simulink model "HydraulicLinearMotorArm"  (R2024a)
settings: Solver=FixedStepAuto  StartTime=0.0  StopTime=inf  MaxStep=0.033333333333333333  RelTol=1e-3  EnableMultiTasking=on
libraries: arduinolib x9, SignalEditorBlockLib x6, arduinosensorlib x2, simulink_extras x1, aerolibanimutils x1
settings Model: ExtModeTrigDuration=2  Creator=Akbar  LastModifiedBy=Akbar
settings SolverCC: AutoInsertRateTranBlk=on
settings OptimizationCC: EnhancedBackFolding=on  PassReuseOutputArgsAs=Individual arguments  ZeroExternalMemoryAtStartup=off  ZeroInternalMemoryAtStartup=off  MaxStackSize=64  OptimizeBlockOrder=speed  DifferentSizesBufferReuse=on  OptimizationCustomize=off  EfficientTunableParamExpr=on
settings DebuggingCC: ParameterTunabilityLossMsg=error
settings HardwareCC: ProdBitPerPointer=32  ProdBitPerSizeT=32  ProdBitPerPtrDiffT=32  ProdLargestAtomicInteger=Long  ProdLargestAtomicFloat=Double  ProdWordSize=32  ProdHWDeviceType=ARM Compatible->ARM Cortex
settings SFSimCC: MATLABDynamicMemAlloc=off
settings RTWCC: Description=Embedded Coder  SystemTargetFile=ert.tlc  HardwareBoard=ESP32-WROOM(Arduino Compatible)  TLCOptions="-aInlineSetEventsForThisBaseRateFcn=TLC_FALSE -aSuppressMultiTaskScheduler=TLC_FALSE  -aRateBasedStepFcn=0"  TemplateMakefile=ert_default_tmf  Toolchain=ESP32  BuildConfiguration=Faster Runs
settings CodeAppCC: ForceParamTrailComments=on  IgnoreCustomStorageClasses=off  OperatorAnnotations=on  SimulinkDataObjDesc=on  SFDataObjDesc=on  InsertBlockDesc=on
settings ERTTargetCC: SupportContinuousTime=on  SupportVariableSizeSignals=on  ExtModeTransport=3  ExtModeStaticAlloc=on  ExtModeAutomaticAllocSize=off  ExtModeStaticAllocSize=65536  ExtModeMexFile=ext_xcp  ExtModeIntrfLevel=Level2 - Open

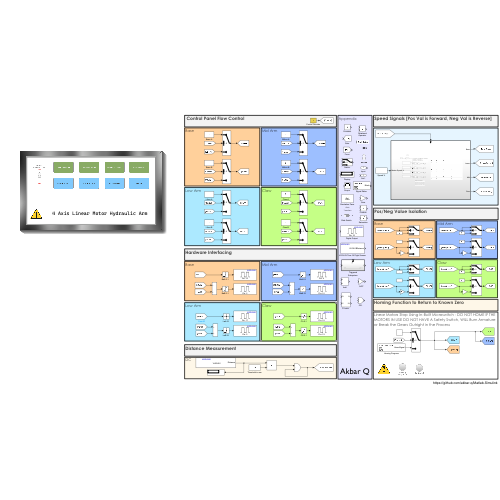
[thumbnail: Simulink's stored preview of the top-level diagram]
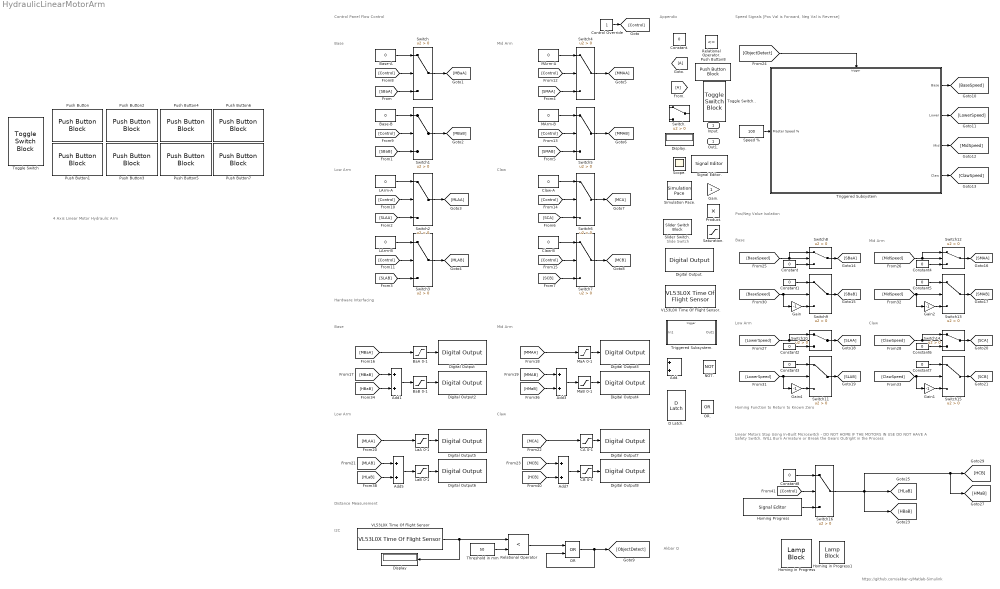
== system HydraulicLinearMotorArm ==
  note: https://github.com/akbar-q/Matlab-Simulink
  note: Akbar Q
  note: 4 Axis Linear Motor Hydraulic Arm
  note: Slide Switch
  note: Appendix
  note: Control Panel Flow Control
  note: Base
  note: Low Arm
  note: Mid Arm
  note: Claw
  note: Claw
  note: Hardware Interfacing
  note: Low Arm
  note: Mid Arm
  note: Base
  note: Distance Measurement
  note: I2C
  note: Speed Signals [Pos Val is Forward, Neg Val is Reverse]
  note: Pos/Neg Value Isolation
  note: Claw
  note: Base
  note: Low Arm
  note: Mid Arm
  note: Homing Function to Return to Known Zero
  note: Linear Motors Stop Using In-Built Microswitch - DO NOT HOME IF THE
      | MOTORS IN USE DO NOT HAVE A Safety Switch, WILL Burn Armature
      | or Break the Gears Outright in the Process
  Input. : Inport
  Add. : Sum
  Add{1,3,5,7} (4 alike) : Sum
  BaA 0-1 : Saturate  UpperLimit=1  LowerLimit=0
  BaB 0-1 : Saturate  UpperLimit=1  LowerLimit=0
  Base-A : Constant  Value=0
  Base-B : Constant  Value=0
  CA 0-1 : Saturate  UpperLimit=1  LowerLimit=0
  CB 0-1 : Saturate  UpperLimit=1  LowerLimit=0
  Claw-A : Constant  Value=0
  Claw-B : Constant  Value=0
  Constant{,1..8} (9 alike) : Constant  Value=0
  Constant. : Constant  Value=0
  Control Override : Constant
  D Latch. : simulink_extras/Flip Flops/D Latch
  Digital Output : arduinolib/Digital Output  pinNumber=15  Direction=output  blockPlatform=arduino
  Digital Output. : arduinolib/Digital Output  pinNumber=33  Direction=output  blockPlatform=arduino
  Digital Output2 : arduinolib/Digital Output  pinNumber=2  Direction=output  blockPlatform=arduino
  Digital Output3 : arduinolib/Digital Output  pinNumber=4  Direction=output  blockPlatform=arduino
  Digital Output4 : arduinolib/Digital Output  pinNumber=16  Direction=output  blockPlatform=arduino
  Digital Output5 : arduinolib/Digital Output  pinNumber=17  Direction=output  blockPlatform=arduino
  Digital Output6 : arduinolib/Digital Output  pinNumber=5  Direction=output  blockPlatform=arduino
  Digital Output7 : arduinolib/Digital Output  pinNumber=18  Direction=output  blockPlatform=arduino
  Digital Output8 : arduinolib/Digital Output  pinNumber=19  Direction=output  blockPlatform=arduino
  Display : Display
  Display. : Display
  From. : From
  Gain{,1..2,4} (4 alike) : Gain  Gain=-1
  Gain. : Gain
  Goto. : Goto
  Homing Progress : SignalEditorBlockLib/Signal Editor  FileName=C:\Users\Akbar\Cloud-Drive_maa32ocd@bolton.ac.uk\Hobby Projects\GitHub Repos\Matlab-Simulink\ESP32-Arm-4DOF-Binary\SpeedSignals\HomeSignal.mat  ActiveScenario=HomingFunction  ActiveSignal=HomeSignal  IsBus=off  OutputBusObjectStr=Bus: BusObject  SampleTime=0  Interpolate=off  ZeroCross=off  OutputAfterFinalValue=Setting to zero  Unit=inherit  PreserveSignalName=on  ApplySigPropsToAllScenarios=on  ApplySigPropsToAllSignals=off
  Homing in Progress : LampBlock  LabelPosition=Bottom
  Homing in Progress1 : LampBlock  LabelPosition=Bottom
  LArm-A : Constant  Value=0
  LArm-B : Constant  Value=0
  LaA 0-1 : Saturate  UpperLimit=1  LowerLimit=0
  LaB 0-1 : Saturate  UpperLimit=1  LowerLimit=0
  MArm-A : Constant  Value=0
  MArm-B : Constant  Value=0
  MaA 0-1 : Saturate  UpperLimit=1  LowerLimit=0
  MaB 0-1 : Saturate  UpperLimit=1  LowerLimit=0
  NOT. : Logic  Operator=NOT  IconShape=distinctive  AllPortsSameDT=off  OutDataTypeStr=boolean
  OR : Logic  Operator=OR  IconShape=distinctive  AllPortsSameDT=off  OutDataTypeStr=boolean
  OR. : Logic  Operator=OR  IconShape=distinctive  AllPortsSameDT=off  OutDataTypeStr=boolean
  Product. : Product
  Push Button : PushButtonBlock  ButtonText=Base Clockwise  OffValue=0.000000
  Push Button1 : PushButtonBlock  ButtonText=Base AntiClock  OffValue=0.000000
  Push Button2 : PushButtonBlock  ButtonText=Low Arm Forward  OffValue=0.000000
  Push Button3 : PushButtonBlock  ButtonText=Low Arm Back  OffValue=0.000000
  Push Button4 : PushButtonBlock  ButtonText=Mid Arm Forward  OffValue=0.000000
  Push Button5 : PushButtonBlock  ButtonText=Mid Arm Back  OffValue=0.000000
  Push Button6 : PushButtonBlock  ButtonText=Claw Forward  OffValue=0.000000
  Push Button7 : PushButtonBlock  ButtonText=Claw Back  OffValue=0.000000
  Push Button8 : PushButtonBlock  ButtonText=Push Button
  Relational Operator : RelationalOperator  Operator=<  OutDataTypeStr=boolean  RndMeth=Simplest  InputSameDT=off
  Relational Operator. : RelationalOperator  Operator=<=  OutDataTypeStr=boolean  RndMeth=Simplest  InputSameDT=off
  Saturation. : Saturate
  Scope. : Scope
  Signal Editor. : SignalEditorBlockLib/Signal Editor  FileName=C:\Users\Akbar\Cloud-Drive_maa32ocd@bolton.ac.uk\Hobby Projects\GitHub Repos\Matlab-Simulink\ESP32-Arm-4DOF-Binary\SpeedSignals\BlankAppendix.mat  ActiveScenario=Scenario  ActiveSignal=Blank  IsBus=off  OutputBusObjectStr=Bus: BusObject  SampleTime=0  Interpolate=off  ZeroCross=off  OutputAfterFinalValue=Setting to zero  Unit=inherit  PreserveSignalName=on  ApplySigPropsToAllScenarios=on  ApplySigPropsToAllSignals=off
  Simulation Pace. : aerolibanimutils/Simulation Pace  SimulationPace=1  SleepMode=Auto  OutputPaceError=off  SampleTime=1/30
  Slider Switch. : SliderSwitchBlock  LabelPosition=Hide
      settings: Values={{'Off', 'On'}, [0 1]}
  Speed % : Constant  Value=100
  Switch{,1..16} (17 alike) : Switch  Criteria=u2 > Threshold  SaturateOnIntegerOverflow=off  InputSameDT=off
  Switch. : Switch  Criteria=u2 > Threshold  SaturateOnIntegerOverflow=off  InputSameDT=off
  Threshold in mm : Constant  Value=50
  Toggle Switch : ToggleSwitchBlock
      settings: Values={{'Off', 'On'}, [0 1]}
  Toggle Switch.. : ToggleSwitchBlock  LabelPosition=Hide
      settings: Values={{'Switch', 'Toggle'}, [0 1]}
  Triggered Subsystem : Subsystem  TreatAsAtomicUnit=on
  Triggered Subsystem. : Subsystem  TreatAsAtomicUnit=on
  VL53L0X Time Of Flight Sensor : arduinosensorlib/VL53L0X Time Of Flight Sensor  I2CModule=0  I2CAddress=0x29  BitRate=1000000  RangingMode=Default  SampleTime=-1
  VL53L0X Time Of Flight Sensor. : arduinosensorlib/VL53L0X Time Of Flight Sensor  I2CModule=0  I2CAddress=0xF  BitRate=1000000  RangingMode=Default  SampleTime=-1
  Out1. : Outport
  wires:
  Base-A/1 -> Switch/1
  Base-B/1 -> Switch1/1
  LArm-A/1 -> Switch2/1
  LArm-B/1 -> Switch3/1
  [SBaA] -> Switch/3
  [SBaB] -> Switch1/3
  [SLAA] -> Switch2/3
  [SLAB] -> Switch3/3
  MArm-B/1 -> Switch5/1
  MArm-A/1 -> Switch4/1
  [SMAA] -> Switch4/3
  [SMAB] -> Switch5/3
  Claw-B/1 -> Switch7/1
  [SCA] -> Switch6/3
  [SCB] -> Switch7/3
  Claw-A/1 -> Switch6/1
  Control Override/1 -> [Control]
  [Control] -> Switch/2
  [Control] -> Switch1/2
  [Control] -> Switch2/2
  [Control] -> Switch3/2
  [Control] -> Switch4/2
  [Control] -> Switch5/2
  [Control] -> Switch6/2
  [Control] -> Switch7/2
  Switch/1 -> [MBaA]
  Switch1/1 -> [MBaB]
  Switch2/1 -> [MLAA]
  Switch3/1 -> [MLAB]
  Switch4/1 -> [MMAA]
  Switch5/1 -> [MMAB]
  Switch6/1 -> [MCA]
  Switch7/1 -> [MCB]
  VL53L0X Time Of Flight Sensor/1 -> Display/1, Relational Operator/1
  Threshold in mm/1 -> Relational Operator/2
  Speed %/1 -> Triggered Subsystem/1(Master Speed %)
  Triggered Subsystem/1(Base) -> [BaseSpeed]
  Triggered Subsystem/2(Lower) -> [LowerSpeed]
  Triggered Subsystem/3(Mid) -> [MidSpeed]
  Triggered Subsystem/4(Claw) -> [ClawSpeed]
  [ObjectDetect] -> Triggered Subsystem/Trigger
  Switch11/1 -> [SLAB]
  [BaseSpeed] -> Switch8/1, Switch8/2
  Switch8/1 -> [SBaA]
  Switch9/1 -> [SBaB]
  [BaseSpeed] -> Gain/1, Switch9/2
  Gain/1 -> Switch9/3
  Constant/1 -> Switch8/3
  Constant1/1 -> Switch9/1
  [MBaA] -> BaA 0-1/1
  [MBaB] -> Add1/1
  [HBaB] -> Add1/2
  BaB 0-1/1 -> Digital Output2/1
  Add1/1 -> BaB 0-1/1
  Constant2/1 -> Switch10/3
  [LowerSpeed] -> Gain4/1, Switch11/2
  Constant3/1 -> Switch11/1
  Gain4/1 -> Switch11/3
  [LowerSpeed] -> Switch10/2, Switch10/1
  Switch10/1 -> [SLAA]
  Switch13/1 -> [SMAB]
  Constant4/1 -> Switch12/3
  Gain2/1 -> Switch13/3
  [MidSpeed] -> Gain2/1, Switch13/2
  Constant5/1 -> Switch13/1
  [MidSpeed] -> Switch12/1, Switch12/2
  Switch12/1 -> [SMAA]
  [ClawSpeed] -> Switch14/1, Switch14/2
  Constant7/1 -> Switch15/1
  Gain1/1 -> Switch15/3
  [ClawSpeed] -> Switch15/2, Gain1/1
  Constant6/1 -> Switch14/3
  Switch14/1 -> [SCA]
  Switch15/1 -> [SCB]
  [HMaB] -> Add3/2
  MaB 0-1/1 -> Digital Output4/1
  MaA 0-1/1 -> Digital Output3/1
  [MMAA] -> MaA 0-1/1
  Add3/1 -> MaB 0-1/1
  [MMAB] -> Add3/1
  LaB 0-1/1 -> Digital Output6/1
  [HLaB] -> Add5/2
  LaA 0-1/1 -> Digital Output5/1
  [MLAA] -> LaA 0-1/1
  Add5/1 -> LaB 0-1/1
  [MLAB] -> Add5/1
  CA 0-1/1 -> Digital Output7/1
  Add7/1 -> CB 0-1/1
  [MCA] -> CA 0-1/1
  [MCB] -> Add7/1
  [HCB] -> Add7/2
  CB 0-1/1 -> Digital Output8/1
  BaA 0-1/1 -> Digital Output/1
  [Control] -> Switch16/2
  Switch16/1 -> [HMaB], [HCB], [HBaB], [HLaB]
  Constant8/1 -> Switch16/1
  Homing Progress/1 -> Switch16/3
  OR/1 -> OR/2, [ObjectDetect]
  Relational Operator/1 -> OR/1

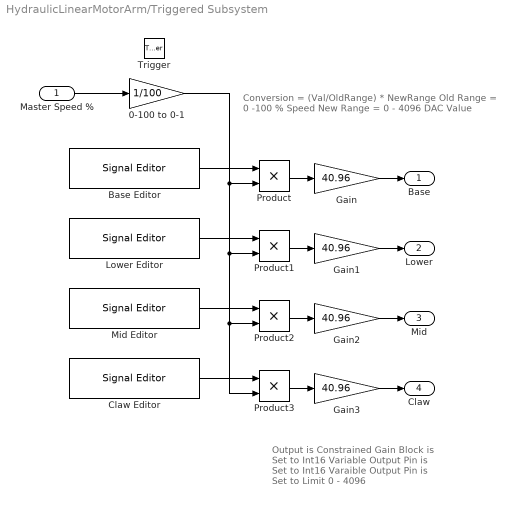
== system HydraulicLinearMotorArm/Triggered Subsystem ==
  note: Conversion = (Val/OldRange) * NewRange
      |
      | Old Range = 0 -100 % Speed
      | New Range = 0 - 4096 DAC Value
  note: Output is Constrained
      |
      | Gain Block is Set to Int16 Variable
      | Output Pin is Set to Int16 Varaible
      | Output Pin is Set to Limit 0 - 4096
  Master Speed % : Inport
  Trigger : TriggerPort  VariantControl=(inherit)
  0-100 to 0-1 : Gain  Gain=1/100
  Base Editor : SignalEditorBlockLib/Signal Editor  FileName=C:\Users\Akbar\Cloud-Drive_maa32ocd@bolton.ac.uk\Hobby Projects\GitHub Repos\Matlab-Simulink\ESP32-Arm-4DOF-Binary\SpeedSignals\BaseSignal.mat  ActiveScenario=PathPlan  ActiveSignal=BaseSignal  IsBus=off  OutputBusObjectStr=Bus: BusObject  SampleTime=-1  ZeroCross=off  OutputAfterFinalValue=Setting to zero  Unit=inherit  PreserveSignalName=on  ApplySigPropsToAllScenarios=on  ApplySigPropsToAllSignals=off
  Claw Editor : SignalEditorBlockLib/Signal Editor  FileName=C:\Users\Akbar\Cloud-Drive_maa32ocd@bolton.ac.uk\Hobby Projects\GitHub Repos\Matlab-Simulink\ESP32-Arm-4DOF-Binary\SpeedSignals\ClawSignal.mat  ActiveScenario=PathPlan  ActiveSignal=ClawSignal  IsBus=off  OutputBusObjectStr=Bus: BusObject  SampleTime=-1  ZeroCross=off  OutputAfterFinalValue=Setting to zero  Unit=inherit  PreserveSignalName=on  ApplySigPropsToAllScenarios=on  ApplySigPropsToAllSignals=off
  Gain{,1..3} (4 alike) : Gain  Gain=40.96  OutDataTypeStr=int16
  Lower Editor : SignalEditorBlockLib/Signal Editor  FileName=C:\Users\Akbar\Cloud-Drive_maa32ocd@bolton.ac.uk\Hobby Projects\GitHub Repos\Matlab-Simulink\ESP32-Arm-4DOF-Binary\SpeedSignals\LowerSignal.mat  ActiveScenario=PathPlan  ActiveSignal=LowerSignal  IsBus=off  OutputBusObjectStr=Bus: BusObject  SampleTime=-1  ZeroCross=off  OutputAfterFinalValue=Setting to zero  Unit=inherit  PreserveSignalName=on  ApplySigPropsToAllScenarios=on  ApplySigPropsToAllSignals=off
  Mid Editor : SignalEditorBlockLib/Signal Editor  FileName=C:\Users\Akbar\Cloud-Drive_maa32ocd@bolton.ac.uk\Hobby Projects\GitHub Repos\Matlab-Simulink\ESP32-Arm-4DOF-Binary\SpeedSignals\MidSignal.mat  ActiveScenario=PathPlan  ActiveSignal=MidSignal  IsBus=off  OutputBusObjectStr=Bus: BusObject  SampleTime=-1  ZeroCross=off  OutputAfterFinalValue=Setting to zero  Unit=inherit  PreserveSignalName=on  ApplySigPropsToAllScenarios=on  ApplySigPropsToAllSignals=off
  Product{,1..3} (4 alike) : Product
  Base : Outport  OutMin=[0]  OutMax=[4096]  OutDataTypeStr=int16
  Lower : Outport  Port=2  OutMin=[0]  OutMax=[4096]  OutDataTypeStr=int16
  Mid : Outport  Port=3  OutMin=[0]  OutMax=[4096]  OutDataTypeStr=int16
  Claw : Outport  Port=4  OutMin=[0]  OutMax=[4096]  OutDataTypeStr=int16
  wires:
  Master Speed %/1 -> 0-100 to 0-1/1
  Base Editor/1 -> Product/1
  Lower Editor/1 -> Product1/1
  Mid Editor/1 -> Product2/1
  Claw Editor/1 -> Product3/1
  Product/1 -> Gain/1
  Product1/1 -> Gain1/1
  Product2/1 -> Gain2/1
  Product3/1 -> Gain3/1
  0-100 to 0-1/1 -> Product/2, Product1/2, Product2/2, Product3/2
  Gain/1 -> Base/1
  Gain1/1 -> Lower/1
  Gain2/1 -> Mid/1
  Gain3/1 -> Claw/1

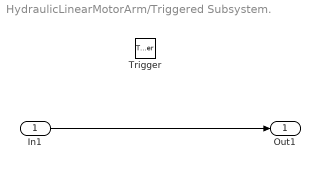
== system HydraulicLinearMotorArm/Triggered Subsystem. ==
  In1 : Inport
  Trigger : TriggerPort  VariantControl=(inherit)
  Out1 : Outport
  wires:
  In1/1 -> Out1/1
